simulink model "FOC_PMSM_FVSensorNew"  (R2019b)
settings: Solver=ode45  StartTime=0  StopTime=1  FixedStep=1/fs/4  MaxStep=1/fs/2  RelTol=1e-7  EnableMultiTasking=on
InitFcn:
  | Motor_parameters_Lsrpm7fw
values from neighbouring files (symbols this model uses):
  c2 = -L2/(L1^2-L2^2)    (= 10.9375)    [Motor_parameters_Lsrpm7fw.m]
  fs = 20e3    (= 20000)    [Motor_parameters_Lsrpm7fw.m]
  Iphmax = I_rated*sqrt(2)*3    [Motor_parameters_Lsrpm7fw.m]
  J = 1*1e-3    (= 0.001)    [Motor_parameters_Lsrpm7fw.m]
  Ki1 = 2    [Motor_parameters_Lsrpm7fw.m]
  Ki2 = 3000    [Motor_parameters_Lsrpm7fw.m]
  Ki_pll = Bw^2*(1.1-0.334*zeta)^2*1/(2*k1)    (= 1705731.55439)    [Motor_parameters_Lsrpm7fw.m]
  Kp1 = 0.005    [Motor_parameters_Lsrpm7fw.m]
  Kp2 = 2    [Motor_parameters_Lsrpm7fw.m]
  Kp_pll = Bw*(2.2*zeta-0.668*zeta^2)*1/(2*k1)    (= 27920.01984)    [Motor_parameters_Lsrpm7fw.m]
  Ld = 10e-3    (= 0.01)    [Motor_parameters_Lsrpm7fw.m]
  Lndd_ini = Lndmpm    (= 0.412)    [Motor_parameters_Lsrpm7fw.m]
  Lndmpm = 0.412    [Motor_parameters_Lsrpm7fw.m]
  Lq = 12.8e-3    (= 0.0128)    [Motor_parameters_Lsrpm7fw.m]
  Npp = 8/2    (= 4)    [Motor_parameters_Lsrpm7fw.m]
  Omegae_ini = 0    [Motor_parameters_Lsrpm7fw.m]
  Rs = 0.78    [Motor_parameters_Lsrpm7fw.m]
  Tl_const = Trat/nrat^2    (= 3.26530612245e-06)    [Motor_parameters_Lsrpm7fw.m]
  Trat = 10    [Motor_parameters_Lsrpm7fw.m]
  Vm = 70    [Motor_parameters_Lsrpm7fw.m]
  Vph = Vs*sqrt(2)    [Motor_parameters_Lsrpm7fw.m]
  wo = 15    [Motor_parameters_Lsrpm7fw.m]
undefined symbols (not defined in the file or in its folder): DiscIntNeverNeededParam, plecs, sigbuilder_block
libraries: simulink x1
(part 2 of 2)

== system FOC_PMSM_FVSensorNew/Position and speed estimation/Triggered Subsystem/abc 2 dq ==
  abc : Inport
  theta : Inport  Port=2
  Mux1 : Mux  Inputs=2
  Mux2 : Mux  Inputs=2
  abc2d : Fcn  Expr=2/3*(u(1)*cos(u(4))+u(2)*cos(u(4)-2*pi/3)+u(3)*cos(u(4)-4*pi/3))
  abc2q : Fcn  Expr=-1*2/3*(u(1)*sin(u(4))+u(2)*sin(u(4)-2*pi/3)+u(3)*sin(u(4)-4*pi/3))
  dq : Outport  VectorParamsAs1DForOutWhenUnconnected=off
  wires:
  Mux2/1 -> dq/1
  abc2q/1 -> Mux2/2
  abc2d/1 -> Mux2/1
  Mux1/1 -> abc2q/1, abc2d/1
  theta/1 -> Mux1/2
  abc/1 -> Mux1/1

== system FOC_PMSM_FVSensorNew/Position and speed estimation/Triggered Subsystem2/abc 2 dq ==
  abc : Inport
  theta : Inport  Port=2
  Mux1 : Mux  Inputs=2
  Mux2 : Mux  Inputs=2
  abc2d : Fcn  Expr=2/3*(u(1)*cos(u(4))+u(2)*cos(u(4)-2*pi/3)+u(3)*cos(u(4)-4*pi/3))
  abc2q : Fcn  Expr=-1*2/3*(u(1)*sin(u(4))+u(2)*sin(u(4)-2*pi/3)+u(3)*sin(u(4)-4*pi/3))
  dq : Outport  VectorParamsAs1DForOutWhenUnconnected=off
  wires:
  Mux2/1 -> dq/1
  abc2q/1 -> Mux2/2
  abc2d/1 -> Mux2/1
  Mux1/1 -> abc2q/1, abc2d/1
  theta/1 -> Mux1/2
  abc/1 -> Mux1/1
